simulink model "Validate_GPIO_Write"  (R2023a)
settings: Solver=FixedStepAuto  StartTime=0.0  StopTime=inf  RelTol=1e-3
undefined symbols (not defined in the file or in its folder): baseRate
libraries: simulink x2
settings Model: Creator=SPOT  LastModifiedBy=alexa
settings OptimizationCC: EnhancedBackFolding=on  PassReuseOutputArgsAs=Individual arguments  ZeroExternalMemoryAtStartup=off  ZeroInternalMemoryAtStartup=off  MaxStackSize=64  OptimizeBlockOrder=speed  DifferentSizesBufferReuse=on  OptimizationCustomize=off  EfficientTunableParamExpr=on
settings DebuggingCC: ParameterTunabilityLossMsg=error
settings HardwareCC: ProdBitPerLong=64  ProdLargestAtomicInteger=LongLong  ProdLargestAtomicFloat=Double  ProdLongLongMode=on  ProdHWDeviceType=ARM Compatible->ARM 64-bit (LP64)
settings SFSimCC: MATLABDynamicMemAlloc=off
settings RTWCC: Description=Embedded Coder  SystemTargetFile=ert.tlc  HardwareBoard=NVIDIA Jetson  TLCOptions="-aInlineSetEventsForThisBaseRateFcn=TLC_FALSE -aSuppressMultiTaskScheduler=TLC_FALSE  -aRateBasedStepFcn=0"  TemplateMakefile=ert_default_tmf
settings CodeAppCC: ForceParamTrailComments=on  IgnoreCustomStorageClasses=off  OperatorAnnotations=on  SimulinkDataObjDesc=on  SFDataObjDesc=on  InsertBlockDesc=on

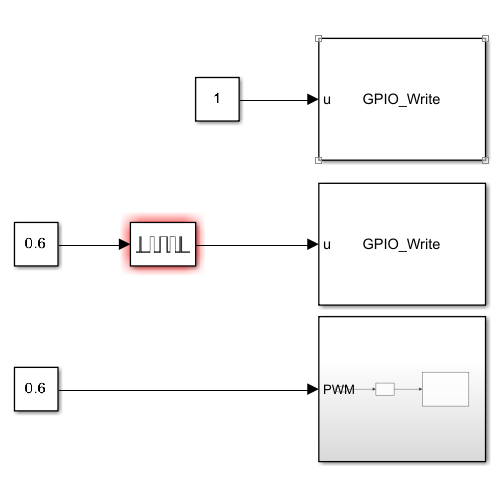
[thumbnail: Simulink's stored preview of the top-level diagram]
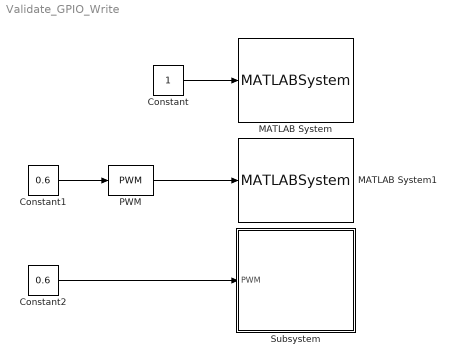
== system Validate_GPIO_Write ==
  Constant : Constant
  Constant1 : Constant  Value=0.6
  Constant2 : Constant  Value=0.6
  MATLAB System : MATLABSystem  System=GPIO_Write  gpioPin=428  pinDirection=1
      mask Type: GPIO_Write
      mask Display:
      | disp('GPIO_Write');
      | port_label('input',1,'u');
  MATLAB System1 : MATLABSystem  System=GPIO_Write  gpioPin=445  pinDirection=1
      mask Type: GPIO_Write
      mask Display:
      | disp('GPIO_Write');
      | port_label('input',1,'u');
  PWM : simulink/Discontinuities/PWM  DisableCoverage=on  Period=0.1  InitialDelay=0  DisallowZeroDutyCycle=off  RunAtFixedTimeIntervals=on  SampleTime=baseRate
  Subsystem : Subsystem
  wires:
  Constant/1 -> MATLAB System/1
  PWM/1 -> MATLAB System1/1
  Constant1/1 -> PWM/1
  Constant2/1 -> Subsystem/1(PWM)

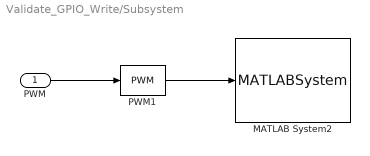
== system Validate_GPIO_Write/Subsystem ==
  PWM : Inport
  MATLAB System2 : MATLABSystem  System=GPIO_Write  gpioPin=480  pinDirection=1
      mask Type: GPIO_Write
      mask Display:
      | disp('GPIO_Write');
      | port_label('input',1,'u');
  PWM1 : simulink/Discontinuities/PWM  DisableCoverage=on  Period=0.1  InitialDelay=0  DisallowZeroDutyCycle=off  RunAtFixedTimeIntervals=on  SampleTime=baseRate
  wires:
  PWM1/1 -> MATLAB System2/1
  PWM/1 -> PWM1/1
